simulink model "EarlyReturn14"  (R2020a)
settings: Solver=VariableStepAuto  StartTime=0.0  StopTime=0.1  RelTol=1e-3
settings Model: Creator=BEAR  LastModifiedBy=bzhan
settings DataIOCC: ReturnWorkspaceOutputs=off
settings DebuggingCC: ArithmeticOperatorsInVariantConditions=warning
settings SFSimCC: SimUseLocalCustomCode=off  CustomCodeUndefinedFunction=UseInterfaceOnly
settings RTWCC: RTWUseLocalCustomCode=off

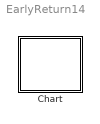
== system EarlyReturn14 ==
  Chart : Stateflow chart  TreatAsAtomicUnit=on

== stateflow chart EarlyReturn14/Chart ==
  settings: updateMethod=DISCRETE  sampleTime=0.1
  state A
    en: f("en_A")
    ex: f("ex_A")
    state A1
      en: f("en_A1")
      ex: f("ex_A1")
    state A2
      en: f("en_A2")
      ex: f("ex_A2")
    (default) -> A1
    A1 -> A2 : {E;f("ca")}/{f("ta")}
  (default) -> A
  A -> A : E{f("loop")}
  data: s function_input
  events: E local FUNCTION_CALL_EVENT
  function f(s):
    | function f(s)
    |   fprintf(s+"\n");
